simulink library "M160_lib"  (Simulink 7.8)
settings: Solver=FixedStepDiscrete  StartTime=0.0  StopTime=10.0  RelTol=1e-3
PreLoadFcn:
  | update_path
undefined symbols (not defined in the file): Afr_atCool2facLambdaReqCorr_CUR_x, Afr_atCool2facLambdaReqCorr_CUR_y, Afr_atMani2facLambdaReqCorr_CUR_x, Afr_atMani2facLambdaReqCorr_CUR_y, Afr_facLambdaReqMan, Afr_facRatioMan, Afr_facStoich, Afr_flgLambdaReqOverride, Afr_flgRatioOverride, Afr_rpmEngSpdfacRelAir2facLambdaReqBase_MAP_x, Afr_rpmEngSpdfacRelAir2facLambdaReqBase_MAP_y, Afr_rpmEngSpdfacRelAir2facLambdaReqBase_MAP_z, Ais_flgAirInjReacPumpOverride, Ais_stAirInjReacPumpMan, Amc_flgAirMassFlowOverride, Amc_uSens2AirMassFlow_CUR_x, Amc_uSens2AirMassFlow_CUR_y, Amc_uSensMaxValid, Amc_uSensMinValid, Amf_facRelAirMan, Amf_flgAirMassPerStrOverride, Amf_flgRelAirOverride, Amf_flgSwitch2AirMassFlowMeter, Amf_mAirPerStrMan, Amf_pManiEngSpd2facRelAirCorr_MAP_x, Amf_pManiEngSpd2facRelAirCorr_MAP_y, Amf_pManiEngSpd2facRelAirCorr_MAP_z, Amf_rpmEngSpd2facTempCorr_CUR_x, Amf_rpmEngSpd2facTempCorr_CUR_y, Amf_shcSpecGasConst_C, Amf_volEngDisp_C, Apv_facAirPumpRateMan, Apv_factor, Apv_flgAirPumpRateOverride, Apv_tiPeriod_C, Bvc_rVoltDivHigh, Bvc_rVoltDivLow, Bvc_uBattMax, Bvc_uBattMin, CDRV_E_OK_, Cov_facChOverVlvRateMan, Cov_factor, Cov_flgChOverVlvRateOverride, Cov_tiPeriod_C, Cpc_atManiTmp2facPresCorr_CUR_x, Cpc_atManiTmp2facPresCorr_CUR_y, Cpc_flgPChargeOverride, Cpc_uSens2pManiBase_CUR_x, Cpc_uSens2pManiBase_CUR_y, Ctc_rPullUp_C, Ctc_rSens2atCool_CUR_x, Ctc_rSens2atCool_CUR_y, Ctc_uSensMaxValid, Ctc_uSensMinValid, Ctc_uSupply, Doh_OutputDiagnosisOverride, dummy_facAirPumpRateReq, dummy_facChOverVlvRateReq, dummy_flgInterCoolerOverride, dummy_flgKl50Override ... (+243)
libraries: simulink x36, ehooks_lib x3
(part 2 of 8)

== system M160_lib/Actuators/Ivc ==
  Opm_idxMode : Inport
  Itc_flgInjCutoff : Inport  Port=2
  Itc_tiInj : Inport  Port=3
  Itc_tiBattDelay : Inport  Port=4
  Ivc : Subsystem
      mask Type: Actuators
      mask Description: InjectionValve
      mask Display:
      | image(imread('InjectionValve.jpg'))
      | port_label('input',1,'Opm_idxMode')
      | port_label('input',2,'Itc_flgInjCutoff')
      | port_label('input',3,'Itc_tiInj')
      | port_label('input',4,'Itc_tiBattDelay')
      | port_label('output',1,'Ivc_flgError')
  Ivc_Diag : Subsystem
      mask Type: Actuators
      mask Description: InjectionValveDiagnose
      mask Display:
      | image(imread('InjectionValve.jpg'))
      | port_label('output',1,'Ivc_flgError')
  Ivc_Diag_set : ehooks_lib/Library Blocks/ECU_FcnCallTrigger_Source  Tag=ECU_FcnCallTrigger_Source  Description=|  ProcessName=BypEasyhooks_100ms_Pre_Proc  TaskPriority=0  TaskPeriod=1
      | [$SL_INT_DD 20060]
      | EHOOKS ECU asynchronous function-call trigger source block.
  Ivc_Error : Subsystem
      mask Type: Actuators
      mask Description: InjectionValveError
      mask Display:
      | image(imread('InjectionValve.jpg'))
      | port_label('output',1,'Ivc_flgError')
  Ivc_set : ehooks_lib/Library Blocks/ECU_FcnCallTrigger_Source  Tag=ECU_FcnCallTrigger_Source  Description=|  ProcessName=BypEasyhooks_S0_Pre_Proc  TaskPriority=0  TaskPeriod=1
      | [$SL_INT_DD 20060]
      | EHOOKS ECU asynchronous function-call trigger source block.
  Ivc_set_Error : ehooks_lib/Library Blocks/ECU_FcnCallTrigger_Source  Tag=ECU_FcnCallTrigger_Source  Description=|  ProcessName=BypEasyhooks_S0_Pre_Proc  TaskPriority=0  TaskPeriod=1
      | [$SL_INT_DD 20060]
      | EHOOKS ECU asynchronous function-call trigger source block.
  Ivc_flgError : Outport
  wires:
  Ivc_set/1 -> Ivc/Trigger
  Ivc_Diag_set/1 -> Ivc_Diag/Trigger
  Opm_idxMode/1 -> Ivc/1(Opm_idxMode)
  Itc_flgInjCutoff/1 -> Ivc/2(Itc_flgInjCutoff)
  Itc_tiInj/1 -> Ivc/3(Itc_tiInj)
  Itc_tiBattDelay/1 -> Ivc/4(Itc_tiBattDelay)
  Ivc_set_Error/1 -> Ivc_Error/Trigger
  Ivc/1(Ivc_flgError) -> Ivc_Error/1(Ivc)
  Ivc_Diag/1(Ivc_flgError) -> Ivc_Error/2(Ivc_Diag)
  Ivc_Error/1(Ivc_flgError) -> Ivc_flgError/1

== system M160_lib/Actuators/Mrs ==
  Opm_idxMode : Inport
  dummy_stMainRelais : Inport  Port=2
  function : TriggerPort  TriggerType=function-call
  Constant1 : Constant  Value=Mrs_flgMainRelaisOverride
  Constant2 : Constant  Value=Mrs_stMainRelaisMan
  Constant5 : Constant  Value=Normal
  Constant6 : Constant  OutDataTypeStr=boolean
  G1_DigOut_Ctrl : Subsystem  AncestorBlock=ehooks_medc17flex_G1_lib/Library Blocks/Basic_IO/Outputs/G1_DigOut_Ctrl  LoadFcn=ehooks_medc17flex_devlib_io_block('load');  InitFcn=ehooks_medc17flex_devlib_io_block('init');  StartFcn=ehooks_medc17flex_devlib_io_block('start');  StopFcn=ehooks_medc17flex_devlib_io_block('stop');  ClipboardFcn=ehooks_medc17flex_devlib_io_block('clipboard', 0); % Second argument just needed to indicate null block. See callback handler.  mask{ChannelName=O_S_MRLY}
      mask prompts: ChannelName "Channel name"
      mask init:
      | ehooks_medc17flex_devlib_io_block('mask_init');
      settings: AttributesFormatString=Channel name: '%<ChannelName>'  CopyFcn=ehooks_medc17flex_devlib_io_block('copy');  DeleteFcn=ehooks_medc17flex_devlib_io_block('delete');  UndoDeleteFcn=ehooks_medc17flex_devlib_io_block('undo_delete');  ModelCloseFcn=ehooks_medc17flex_devlib_io_block('model_close');  PreSaveFcn=ehooks_medc17flex_devlib_io_block('pre_save');  PostSaveFcn=ehooks_medc17flex_devlib_io_block('post_save');  NameChangeFcn=ehooks_medc17flex_devlib_io_block('name_change');  DestroyFcn=ehooks_medc17flex_devlib_io_block('destroy', 0); % Second argument just needed to indicate null block. See callback handler.  OpenFcn=ehooks_medc17flex_devlib_io_block('open');  CloseFcn=ehooks_medc17flex_devlib_io_block('close');  ParentCloseFcn=ehooks_medc17flex_devlib_io_block('parent_close');  MoveFcn=ehooks_medc17flex_devlib_io_block('move');
      mask StyleString: popup(<empty>|O_S_MRLY|O_S_RL09|O_S_RL14|O_S_RL29|O_S_RL30|O_S_RL31|O_S_RL33|O_S_RL34|O_S_RL35|O_S_RL41|O_S_RL43)
      mask Display: image(imread('Output_Digital.jpg'))
  G1_DigOut_GetError : Subsystem  AncestorBlock=ehooks_medc17flex_G1_lib/Library Blocks/Basic_IO/Outputs/G1_DigOut_GetError  LoadFcn=ehooks_medc17flex_devlib_io_block('load');  InitFcn=ehooks_medc17flex_devlib_io_block('init');  StartFcn=ehooks_medc17flex_devlib_io_block('start');  StopFcn=ehooks_medc17flex_devlib_io_block('stop');  ClipboardFcn=ehooks_medc17flex_devlib_io_block('clipboard', 0); % Second argument just needed to indicate null block. See callback handler.  mask{ChannelName=O_S_MRLY}
      mask prompts: ChannelName "Channel name"
      mask init:
      | ehooks_medc17flex_devlib_io_block('mask_init');
      settings: AttributesFormatString=Channel name: '%<ChannelName>'  CopyFcn=ehooks_medc17flex_devlib_io_block('copy');  DeleteFcn=ehooks_medc17flex_devlib_io_block('delete');  UndoDeleteFcn=ehooks_medc17flex_devlib_io_block('undo_delete');  ModelCloseFcn=ehooks_medc17flex_devlib_io_block('model_close');  PreSaveFcn=ehooks_medc17flex_devlib_io_block('pre_save');  PostSaveFcn=ehooks_medc17flex_devlib_io_block('post_save');  NameChangeFcn=ehooks_medc17flex_devlib_io_block('name_change');  DestroyFcn=ehooks_medc17flex_devlib_io_block('destroy', 0); % Second argument just needed to indicate null block. See callback handler.  OpenFcn=ehooks_medc17flex_devlib_io_block('open');  CloseFcn=ehooks_medc17flex_devlib_io_block('close');  ParentCloseFcn=ehooks_medc17flex_devlib_io_block('parent_close');  MoveFcn=ehooks_medc17flex_devlib_io_block('move');
      mask StyleString: popup(<empty>|O_S_MRLY|O_S_RL09|O_S_RL14|O_S_RL29|O_S_RL30|O_S_RL31|O_S_RL33|O_S_RL34|O_S_RL35|O_S_RL41|O_S_RL43)
      mask Display: image(imread('Output_Digital_Diagnosis.jpg'))
  Logical Operator1 : Logic  Operator=NOT  AllPortsSameDT=off  OutDataTypeStr=boolean
  Logical Operator2 : Logic  Operator=NOT  AllPortsSameDT=off  OutDataTypeStr=boolean
  Relational Operator : RelationalOperator  Operator===  OutDataTypeStr=boolean
  Switch1 : Switch  Threshold=1
  Switch2 : Switch  Threshold=1
  Mrs_stDiagnosis : Outport
  Mrs_flgError : Outport  Port=2
  wires:
  Constant6/1 -> Switch2/3
  Relational Operator/1 -> Switch2/2
  Constant5/1 -> Relational Operator/2
  Opm_idxMode/1 -> Relational Operator/1
  Switch1/1 -> Switch2/1
  dummy_stMainRelais/1 -> Switch1/3
  Constant2/1 -> Switch1/1
  Constant1/1 -> Switch1/2
  Logical Operator1/1 -> Mrs_flgError/1  "Mrs_flgError"
  G1_DigOut_GetError/1(status) -> Mrs_stDiagnosis/1  "Mrs_stDiagnosis"
  Switch2/1 -> Logical Operator2/1  "Mrs_stMainRelais"
  Logical Operator2/1 -> G1_DigOut_Ctrl/1(state)
  G1_DigOut_Ctrl/1(status) -> Logical Operator1/1

== system M160_lib/Actuators/Str ==
  Opm_idxMode : Inport
  Stc_stStarter : Inport  Port=2
  function : TriggerPort  TriggerType=function-call
  Constant1 : Constant  Value=Str_flgStarterOverride
  Constant2 : Constant  Value=Str_stStarterMan
  Constant5 : Constant  Value=Normal
  Constant6 : Constant  Value=0  OutDataTypeStr=boolean
  G1_DigOut_Ctrl : Subsystem  AncestorBlock=ehooks_medc17flex_G1_lib/Library Blocks/Basic_IO/Outputs/G1_DigOut_Ctrl  LoadFcn=ehooks_medc17flex_devlib_io_block('load');  InitFcn=ehooks_medc17flex_devlib_io_block('init');  StartFcn=ehooks_medc17flex_devlib_io_block('start');  StopFcn=ehooks_medc17flex_devlib_io_block('stop');  ClipboardFcn=ehooks_medc17flex_devlib_io_block('clipboard', 0); % Second argument just needed to indicate null block. See callback handler.  mask{ChannelName=O_S_RL34}
      mask prompts: ChannelName "Channel name"
      mask init:
      | ehooks_medc17flex_devlib_io_block('mask_init');
      settings: AttributesFormatString=Channel name: '%<ChannelName>'  CopyFcn=ehooks_medc17flex_devlib_io_block('copy');  DeleteFcn=ehooks_medc17flex_devlib_io_block('delete');  UndoDeleteFcn=ehooks_medc17flex_devlib_io_block('undo_delete');  ModelCloseFcn=ehooks_medc17flex_devlib_io_block('model_close');  PreSaveFcn=ehooks_medc17flex_devlib_io_block('pre_save');  PostSaveFcn=ehooks_medc17flex_devlib_io_block('post_save');  NameChangeFcn=ehooks_medc17flex_devlib_io_block('name_change');  DestroyFcn=ehooks_medc17flex_devlib_io_block('destroy', 0); % Second argument just needed to indicate null block. See callback handler.  OpenFcn=ehooks_medc17flex_devlib_io_block('open');  CloseFcn=ehooks_medc17flex_devlib_io_block('close');  ParentCloseFcn=ehooks_medc17flex_devlib_io_block('parent_close');  MoveFcn=ehooks_medc17flex_devlib_io_block('move');
      mask StyleString: popup(<empty>|O_S_MRLY|O_S_RL09|O_S_RL14|O_S_RL29|O_S_RL30|O_S_RL31|O_S_RL33|O_S_RL34|O_S_RL35|O_S_RL41|O_S_RL43)
      mask Display: image(imread('Output_Digital.jpg'))
  G1_DigOut_GetError : Subsystem  AncestorBlock=ehooks_medc17flex_G1_lib/Library Blocks/Basic_IO/Outputs/G1_DigOut_GetError  LoadFcn=ehooks_medc17flex_devlib_io_block('load');  InitFcn=ehooks_medc17flex_devlib_io_block('init');  StartFcn=ehooks_medc17flex_devlib_io_block('start');  StopFcn=ehooks_medc17flex_devlib_io_block('stop');  ClipboardFcn=ehooks_medc17flex_devlib_io_block('clipboard', 0); % Second argument just needed to indicate null block. See callback handler.  mask{ChannelName=O_S_RL34}
      mask prompts: ChannelName "Channel name"
      mask init:
      | ehooks_medc17flex_devlib_io_block('mask_init');
      settings: AttributesFormatString=Channel name: '%<ChannelName>'  CopyFcn=ehooks_medc17flex_devlib_io_block('copy');  DeleteFcn=ehooks_medc17flex_devlib_io_block('delete');  UndoDeleteFcn=ehooks_medc17flex_devlib_io_block('undo_delete');  ModelCloseFcn=ehooks_medc17flex_devlib_io_block('model_close');  PreSaveFcn=ehooks_medc17flex_devlib_io_block('pre_save');  PostSaveFcn=ehooks_medc17flex_devlib_io_block('post_save');  NameChangeFcn=ehooks_medc17flex_devlib_io_block('name_change');  DestroyFcn=ehooks_medc17flex_devlib_io_block('destroy', 0); % Second argument just needed to indicate null block. See callback handler.  OpenFcn=ehooks_medc17flex_devlib_io_block('open');  CloseFcn=ehooks_medc17flex_devlib_io_block('close');  ParentCloseFcn=ehooks_medc17flex_devlib_io_block('parent_close');  MoveFcn=ehooks_medc17flex_devlib_io_block('move');
      mask StyleString: popup(<empty>|O_S_MRLY|O_S_RL09|O_S_RL14|O_S_RL29|O_S_RL30|O_S_RL31|O_S_RL33|O_S_RL34|O_S_RL35|O_S_RL41|O_S_RL43)
      mask Display: image(imread('Output_Digital_Diagnosis.jpg'))
  Logical Operator1 : Logic  Operator=NOT  AllPortsSameDT=off  OutDataTypeStr=boolean
  Logical Operator2 : Logic  Operator=NOT  AllPortsSameDT=off  OutDataTypeStr=boolean
  Relational Operator : RelationalOperator  Operator===  OutDataTypeStr=boolean
  Switch1 : Switch  Threshold=1
  Switch2 : Switch  Threshold=1
  Str_stDiagnosis : Outport
  Str_flgError : Outport  Port=2
  wires:
  Constant6/1 -> Switch2/3
  Relational Operator/1 -> Switch2/2
  Constant5/1 -> Relational Operator/2
  Opm_idxMode/1 -> Relational Operator/1
  Switch1/1 -> Switch2/1
  Stc_stStarter/1 -> Switch1/3
  Constant2/1 -> Switch1/1
  Constant1/1 -> Switch1/2
  Logical Operator1/1 -> Str_flgError/1  "Str_flgError"
  G1_DigOut_GetError/1(status) -> Str_stDiagnosis/1  "Str_stDiagnosis"
  Switch2/1 -> Logical Operator2/1  "Str_stStarter"
  Logical Operator2/1 -> G1_DigOut_Ctrl/1(state)
  G1_DigOut_Ctrl/1(status) -> Logical Operator1/1

== system M160_lib/Actuators/Tvc ==
  Opm_idxMode : Inport
  dummy_facThrValveReq : Inport  Port=2
  function : TriggerPort  TriggerType=function-call
  Bus Creator : BusCreator  Inputs=3
  Bus Selector : BusSelector  OutputSignals=Tvc_flgPosError,Tvc_facThrValveReq,Tvc_facThrValve
  Constant1 : Constant  Value=Tvc_flgThrValveReqOverride
  Constant2 : Constant  Value=Tvc_facThrValveReqMan
  Constant3 : Constant  Value=Tvc_facThrValveLimitMax
  Constant4 : Constant  Value=Tvc_facThrValveLimitMin
  Constant5 : Constant  Value=Normal
  Constant6 : Constant  Value=0.0  OutDataTypeStr=single
  Limiter : Subsystem
      mask Description: Limiter
      mask Display: image(imread('Limiter.jpg'))
  Logical Operator : Logic  Operator=OR  AllPortsSameDT=off  OutDataTypeStr=boolean
  Logical Operator1 : Logic  Operator=NOT  AllPortsSameDT=off  OutDataTypeStr=boolean
  Relational Operator : RelationalOperator  Operator===  OutDataTypeStr=boolean
  Switch1 : Switch  Threshold=1
  Switch2 : Switch  Threshold=1
  ThrottleValveControl : Subsystem
  ThrottleValveOutput : Subsystem
  ThrottleValvePosition : Subsystem
  Tvc_stDiagnosis : Outport
  Tvc_flgError : Outport  Port=2
  tag scope: Opm_idxMode_global=global
  wires:
  ThrottleValvePosition/1(Tvc_flgPosError) -> Bus Creator/1  "Tvc_flgPosError"
  ThrottleValvePosition/2(Tvc_facThrValve) -> Bus Creator/2  "Tvc_facThrValve"
  Bus Creator/1 -> Bus Selector/1
  Bus Selector/1 -> Logical Operator/1, ThrottleValveOutput/1(Tvc_flgPosError), ThrottleValveControl/1(Tvc_flgPosError)  "<Tvc_flgPosError>"
  Logical Operator1/1 -> Logical Operator/2
  ThrottleValveOutput/1(Tvc_stHBridge) -> Logical Operator1/1
  ThrottleValveControl/1(Tvc_facDutycycle) -> ThrottleValveOutput/2(Tvc_facDutycycle)  "Tvc_facDutycycle"
  Constant3/1 -> Limiter/1(max)
  Constant4/1 -> Limiter/3(min)
  dummy_facThrValveReq/1 -> Limiter/2(in)
  Constant1/1 -> Switch1/2
  Opm_idxMode/1 -> [Opm_idxMode_global], Relational Operator/1
  Constant5/1 -> Relational Operator/2
  Relational Operator/1 -> Switch2/2
  Switch1/1 -> Switch2/1
  Switch2/1 -> Bus Creator/3  "Tvc_facThrValveReq"
  Constant6/1 -> Switch2/3
  Logical Operator/1 -> Tvc_flgError/1  "Tvc_flgError"
  Bus Selector/2 -> ThrottleValveControl/2(Tvc_facThrValve)  "<Tvc_facThrValveReq>"
  Bus Selector/3 -> ThrottleValveControl/3(Tvc_facThrValveReq)  "<Tvc_facThrValve>"
  ThrottleValveOutput/2(Tvc_stDiagnosis) -> Tvc_stDiagnosis/1  "Tvc_stDiagnosis"
  Limiter/1(return) -> Switch1/3
  Constant2/1 -> Switch1/1

== system M160_lib/Actuators/Wcs ==
  Opm_idxMode : Inport
  Ctc_atCool : Inport  Port=2
  function : TriggerPort  TriggerType=function-call
  Constant1 : Constant  Value=Wcs_flgWaterCoolerOverride
  Constant2 : Constant  Value=Wcs_stWaterCoolerMan
  Constant5 : Constant  Value=Normal
  Constant6 : Constant  Value=0  OutDataTypeStr=boolean
  G1_DigOut_Ctrl : Subsystem  AncestorBlock=ehooks_medc17flex_G1_lib/Library Blocks/Basic_IO/Outputs/G1_DigOut_Ctrl  LoadFcn=ehooks_medc17flex_devlib_io_block('load');  InitFcn=ehooks_medc17flex_devlib_io_block('init');  StartFcn=ehooks_medc17flex_devlib_io_block('start');  StopFcn=ehooks_medc17flex_devlib_io_block('stop');  ClipboardFcn=ehooks_medc17flex_devlib_io_block('clipboard', 0); % Second argument just needed to indicate null block. See callback handler.  mask{ChannelName=O_S_RL14}
      mask prompts: ChannelName "Channel name"
      mask init:
      | ehooks_medc17flex_devlib_io_block('mask_init');
      settings: AttributesFormatString=Channel name: '%<ChannelName>'  CopyFcn=ehooks_medc17flex_devlib_io_block('copy');  DeleteFcn=ehooks_medc17flex_devlib_io_block('delete');  UndoDeleteFcn=ehooks_medc17flex_devlib_io_block('undo_delete');  ModelCloseFcn=ehooks_medc17flex_devlib_io_block('model_close');  PreSaveFcn=ehooks_medc17flex_devlib_io_block('pre_save');  PostSaveFcn=ehooks_medc17flex_devlib_io_block('post_save');  NameChangeFcn=ehooks_medc17flex_devlib_io_block('name_change');  DestroyFcn=ehooks_medc17flex_devlib_io_block('destroy', 0); % Second argument just needed to indicate null block. See callback handler.  OpenFcn=ehooks_medc17flex_devlib_io_block('open');  CloseFcn=ehooks_medc17flex_devlib_io_block('close');  ParentCloseFcn=ehooks_medc17flex_devlib_io_block('parent_close');  MoveFcn=ehooks_medc17flex_devlib_io_block('move');
      mask StyleString: popup(<empty>|O_S_MRLY|O_S_RL09|O_S_RL14|O_S_RL29|O_S_RL30|O_S_RL31|O_S_RL33|O_S_RL34|O_S_RL35|O_S_RL41|O_S_RL43)
      mask Display: image(imread('Output_Digital.jpg'))
  G1_DigOut_GetError : Subsystem  AncestorBlock=ehooks_medc17flex_G1_lib/Library Blocks/Basic_IO/Outputs/G1_DigOut_GetError  LoadFcn=ehooks_medc17flex_devlib_io_block('load');  InitFcn=ehooks_medc17flex_devlib_io_block('init');  StartFcn=ehooks_medc17flex_devlib_io_block('start');  StopFcn=ehooks_medc17flex_devlib_io_block('stop');  ClipboardFcn=ehooks_medc17flex_devlib_io_block('clipboard', 0); % Second argument just needed to indicate null block. See callback handler.  mask{ChannelName=O_S_RL14}
      mask prompts: ChannelName "Channel name"
      mask init:
      | ehooks_medc17flex_devlib_io_block('mask_init');
      settings: AttributesFormatString=Channel name: '%<ChannelName>'  CopyFcn=ehooks_medc17flex_devlib_io_block('copy');  DeleteFcn=ehooks_medc17flex_devlib_io_block('delete');  UndoDeleteFcn=ehooks_medc17flex_devlib_io_block('undo_delete');  ModelCloseFcn=ehooks_medc17flex_devlib_io_block('model_close');  PreSaveFcn=ehooks_medc17flex_devlib_io_block('pre_save');  PostSaveFcn=ehooks_medc17flex_devlib_io_block('post_save');  NameChangeFcn=ehooks_medc17flex_devlib_io_block('name_change');  DestroyFcn=ehooks_medc17flex_devlib_io_block('destroy', 0); % Second argument just needed to indicate null block. See callback handler.  OpenFcn=ehooks_medc17flex_devlib_io_block('open');  CloseFcn=ehooks_medc17flex_devlib_io_block('close');  ParentCloseFcn=ehooks_medc17flex_devlib_io_block('parent_close');  MoveFcn=ehooks_medc17flex_devlib_io_block('move');
      mask StyleString: popup(<empty>|O_S_MRLY|O_S_RL09|O_S_RL14|O_S_RL29|O_S_RL30|O_S_RL31|O_S_RL33|O_S_RL34|O_S_RL35|O_S_RL41|O_S_RL43)
      mask Display: image(imread('Output_Digital_Diagnosis.jpg'))
  Hysteresis_Delta_RSP : Subsystem
      mask Description: Hysteresis_Delta_RSP
      mask Display: image(imread('HysteresDeltaR.jpg'))
  Logical Operator1 : Logic  Operator=NOT  AllPortsSameDT=off  OutDataTypeStr=boolean
  Logical Operator2 : Logic  Operator=NOT  AllPortsSameDT=off  OutDataTypeStr=boolean
  Relational Operator : RelationalOperator  Operator===  OutDataTypeStr=boolean
  Switch1 : Switch  Threshold=1
  Switch2 : Switch  Threshold=1
  Wcs_stDiagnosis : Outport
  Wcs_flgError : Outport  Port=2
  wires:
  Constant6/1 -> Switch2/3
  Relational Operator/1 -> Switch2/2
  Constant5/1 -> Relational Operator/2
  Opm_idxMode/1 -> Relational Operator/1
  Switch1/1 -> Switch2/1
  Ctc_atCool/1 -> Hysteresis_Delta_RSP/1(in)
  Constant2/1 -> Switch1/1
  Constant1/1 -> Switch1/2
  Logical Operator1/1 -> Wcs_flgError/1  "Wcs_flgError"
  G1_DigOut_GetError/1(status) -> Wcs_stDiagnosis/1  "Wcs_stDiagnosis"
  Switch2/1 -> Logical Operator2/1  "Wcs_stWaterCooler"
  Logical Operator2/1 -> G1_DigOut_Ctrl/1(state)
  G1_DigOut_Ctrl/1(status) -> Logical Operator1/1
  Hysteresis_Delta_RSP/1(return) -> Switch1/3

== system M160_lib/Actuators/Wgc ==
  Opm_idxMode : Inport
  T2t_facWasteGateRate : Inport  Port=2
  function : TriggerPort  TriggerType=function-call
  Constant1 : Constant  Value=Wgc_flgWastegateRateOverride
  Constant2 : Constant  Value=Wgc_facWasteGateRateMan
  Constant3 : Constant  Value=10000  OutDataTypeStr=single
  Constant4 : Constant  Value=Wgc_factor
  Constant5 : Constant  Value=Normal
  Constant6 : Constant  Value=0.0  OutDataTypeStr=single
  Constant7 : Constant  Value=Wgc_tiPeriod_C
  Constant9 : Constant  Value=Lo_
  G1_PWM_Output_Ctrl : Subsystem  AncestorBlock=ehooks_medc17flex_G1_lib/Library Blocks/Basic_IO/Outputs/G1_PWM_Output_Ctrl  LoadFcn=ehooks_medc17flex_devlib_io_block('load');  InitFcn=ehooks_medc17flex_devlib_io_block('init');  StartFcn=ehooks_medc17flex_devlib_io_block('start');  StopFcn=ehooks_medc17flex_devlib_io_block('stop');  ClipboardFcn=ehooks_medc17flex_devlib_io_block('clipboard', 0); % Second argument just needed to indicate null block. See callback handler.  mask{ChannelName=O_T_RL22}
      mask prompts: ChannelName "Channel name"
      mask init:
      | ehooks_medc17flex_devlib_io_block('mask_init');
      settings: AttributesFormatString=Channel name: '%<ChannelName>'  CopyFcn=ehooks_medc17flex_devlib_io_block('copy');  DeleteFcn=ehooks_medc17flex_devlib_io_block('delete');  UndoDeleteFcn=ehooks_medc17flex_devlib_io_block('undo_delete');  ModelCloseFcn=ehooks_medc17flex_devlib_io_block('model_close');  PreSaveFcn=ehooks_medc17flex_devlib_io_block('pre_save');  PostSaveFcn=ehooks_medc17flex_devlib_io_block('post_save');  NameChangeFcn=ehooks_medc17flex_devlib_io_block('name_change');  DestroyFcn=ehooks_medc17flex_devlib_io_block('destroy', 0); % Second argument just needed to indicate null block. See callback handler.  OpenFcn=ehooks_medc17flex_devlib_io_block('open');  CloseFcn=ehooks_medc17flex_devlib_io_block('close');  ParentCloseFcn=ehooks_medc17flex_devlib_io_block('parent_close');  MoveFcn=ehooks_medc17flex_devlib_io_block('move');
      mask StyleString: popup(<empty>|O_T_RL10|O_T_RL13|O_T_RL19|O_T_RL20|O_T_RL22|O_T_RL23|O_T_RL25|O_T_RL26|O_T_RL27|O_T_RL28|O_T_RL38|O_T_RL39|O_T_RL40|O_T_RL42|O_T_RL44|O_T_RL45|O_T_RL46|O_T_RL47|O_T_RL48|O_T_RL49|O_T_RL50|O_T_RH02)
      mask Display: image(imread('Output_PWM.jpg'))
  G1_PwmOut_Get_error : Subsystem  AncestorBlock=ehooks_medc17flex_G1_lib/Library Blocks/Basic_IO/Outputs/G1_PwmOut_Get_error  LoadFcn=ehooks_medc17flex_devlib_io_block('load');  InitFcn=ehooks_medc17flex_devlib_io_block('init');  StartFcn=ehooks_medc17flex_devlib_io_block('start');  StopFcn=ehooks_medc17flex_devlib_io_block('stop');  ClipboardFcn=ehooks_medc17flex_devlib_io_block('clipboard', 0); % Second argument just needed to indicate null block. See callback handler.  mask{ChannelName=O_T_RL22}
      mask prompts: ChannelName "Channel name"
      mask init:
      | ehooks_medc17flex_devlib_io_block('mask_init');
      settings: AttributesFormatString=Channel name: '%<ChannelName>'  CopyFcn=ehooks_medc17flex_devlib_io_block('copy');  DeleteFcn=ehooks_medc17flex_devlib_io_block('delete');  UndoDeleteFcn=ehooks_medc17flex_devlib_io_block('undo_delete');  ModelCloseFcn=ehooks_medc17flex_devlib_io_block('model_close');  PreSaveFcn=ehooks_medc17flex_devlib_io_block('pre_save');  PostSaveFcn=ehooks_medc17flex_devlib_io_block('post_save');  NameChangeFcn=ehooks_medc17flex_devlib_io_block('name_change');  DestroyFcn=ehooks_medc17flex_devlib_io_block('destroy', 0); % Second argument just needed to indicate null block. See callback handler.  OpenFcn=ehooks_medc17flex_devlib_io_block('open');  CloseFcn=ehooks_medc17flex_devlib_io_block('close');  ParentCloseFcn=ehooks_medc17flex_devlib_io_block('parent_close');  MoveFcn=ehooks_medc17flex_devlib_io_block('move');
      mask StyleString: popup(<empty>|O_T_RL10|O_T_RL13|O_T_RL19|O_T_RL20|O_T_RL22|O_T_RL23|O_T_RL25|O_T_RL26|O_T_RL27|O_T_RL28|O_T_RL38|O_T_RL39|O_T_RL40|O_T_RL42|O_T_RL44|O_T_RL45|O_T_RL46|O_T_RL47|O_T_RL48|O_T_RL49|O_T_RL50|O_T_RH02)
      mask Display: image(imread('Output_PWM_Diagnosis.jpg'))
  Logical Operator1 : Logic  Operator=NOT  AllPortsSameDT=off  OutDataTypeStr=boolean
  Product1 : Product  OutDataTypeStr=Inherit: Same as first input
  Relational Operator : RelationalOperator  Operator===  OutDataTypeStr=boolean
  Switch1 : Switch  Threshold=1
  Switch2 : Switch  Threshold=1
  Fps_stDiagnosis : Outport
  Fps_flgError : Outport  Port=2
  wires:
  Constant6/1 -> Switch2/3
  Relational Operator/1 -> Switch2/2
  Constant5/1 -> Relational Operator/2
  Opm_idxMode/1 -> Relational Operator/1
  Switch1/1 -> Switch2/1
  T2t_facWasteGateRate/1 -> Switch1/3
  Constant2/1 -> Switch1/1
  Constant1/1 -> Switch1/2
  Logical Operator1/1 -> Fps_flgError/1  "Wgc_flgError"
  G1_PwmOut_Get_error/1(status) -> Fps_stDiagnosis/1  "Wgc_stDiagnosis"
  Switch2/1 -> Product1/1  "Wgc_facWasteGateRate"
  G1_PWM_Output_Ctrl/1(status) -> Logical Operator1/1
  Constant3/1 -> Product1/2
  Product1/1 -> G1_PWM_Output_Ctrl/1(dutycycle)
  Constant7/1 -> G1_PWM_Output_Ctrl/2(period)
  Constant4/1 -> G1_PWM_Output_Ctrl/3(factor)
  Constant9/1 -> G1_PWM_Output_Ctrl/4(level)

== system M160_lib/Functions/Afr ==
  Epm_rpmEngSpd : Inport
  Mtc_atMani : Inport  Port=2
  Ctc_atCool : Inport  Port=3
  Amf_facRelAir : Inport  Port=4
  function : TriggerPort  TriggerType=function-call
  Afr_atCool2facLambdaReqCorr_CUR : Lookup_n-D  NumberOfTableDimensions=1  BreakpointsForDimension1=Afr_atCool2facLambdaReqCorr_CUR_x  Table=Afr_atCool2facLambdaReqCorr_CUR_y  ExtrapMethod=Clip  InputSameDT=on
  Afr_atMani2facLambdaReqCorr_CUR : Lookup_n-D  NumberOfTableDimensions=1  BreakpointsForDimension1=Afr_atMani2facLambdaReqCorr_CUR_x  Table=Afr_atMani2facLambdaReqCorr_CUR_y  ExtrapMethod=Clip  InputSameDT=on
  Afr_rpmEngSpdfacRelAir2facLambdaReqBase_MAP : Lookup_n-D  BreakpointsForDimension1=Afr_rpmEngSpdfacRelAir2facLambdaReqBase_MAP_x  BreakpointsForDimension2=Afr_rpmEngSpdfacRelAir2facLambdaReqBase_MAP_y  Table=Afr_rpmEngSpdfacRelAir2facLambdaReqBase_MAP_z  ExtrapMethod=Clip  InputSameDT=on
  Constant1 : Constant  Value=Afr_flgLambdaReqOverride
  Constant2 : Constant  Value=Afr_flgRatioOverride
  Constant3 : Constant  Value=Afr_facLambdaReqMan
  Constant4 : Constant  Value=Afr_facRatioMan
  Constant5 : Constant  Value=Afr_facStoich
  Product2 : Product  OutDataTypeStr=Inherit: Same as first input
  Subtract : Sum  OutDataTypeStr=Inherit: Same as first input
  Subtract1 : Sum  OutDataTypeStr=Inherit: Same as first input
  Switch1 : Switch  Threshold=1
  Switch2 : Switch  Threshold=1
  Afr_facLambdaReq : Outport
  Afr_facRatio : Outport  Port=2
  wires:
  Epm_rpmEngSpd/1 -> Afr_rpmEngSpdfacRelAir2facLambdaReqBase_MAP/1
  Amf_facRelAir/1 -> Afr_rpmEngSpdfacRelAir2facLambdaReqBase_MAP/2
  Afr_rpmEngSpdfacRelAir2facLambdaReqBase_MAP/1 -> Subtract/1
  Subtract/1 -> Subtract1/1
  Ctc_atCool/1 -> Afr_atCool2facLambdaReqCorr_CUR/1
  Afr_atCool2facLambdaReqCorr_CUR/1 -> Subtract/2
  Mtc_atMani/1 -> Afr_atMani2facLambdaReqCorr_CUR/1
  Afr_atMani2facLambdaReqCorr_CUR/1 -> Subtract1/2
  Subtract1/1 -> Switch1/3, Product2/1  "Afr_facLambdaReqCalc"
  Constant1/1 -> Switch1/2
  Constant3/1 -> Switch1/1
  Switch1/1 -> Afr_facLambdaReq/1  "Afr_facLambdaReq"
  Switch2/1 -> Afr_facRatio/1  "Afr_facRatio"
  Product2/1 -> Switch2/3  "Afr_facRatioCalc"
  Constant5/1 -> Product2/2
  Constant2/1 -> Switch2/2
  Constant4/1 -> Switch2/1

== system M160_lib/Functions/Amf ==
  note: Pa/(K*(J/(K*kg))) = (N/m^2)/(K*(N*m/(K*kg))) = kg/m^3
  note: cm^3*kg/m^3 = 10^-6*m^3*10^3*g/m^3 = 10^-3*g
  note: 1000 g/kg - Umrechnung in kg
      | 2 - 2 Umdrehungen pro Arbeitsspiel
  note: umrechung Drehzahl in 1/h
  note: 1000 g/kg - Umrechnung in kg
      | 2 - 2 Umdrehungen pro Arbeitsspiel
  Epm_rpmEngSpd : Inport
  Mtc_atMani : Inport  Port=2
  Mpc_pManiFilt : Inport  Port=3
  Ctc_atCool : Inport  Port=4
  Amc_AirMassFlow : Inport  Port=5
  function : TriggerPort  TriggerType=function-call
  Amf_mAirCalc : Terminator
  Amf_pManiEngSpd2facRelAirCorr_MAP : Lookup_n-D  BreakpointsForDimension1=Amf_pManiEngSpd2facRelAirCorr_MAP_x  BreakpointsForDimension2=Amf_pManiEngSpd2facRelAirCorr_MAP_y  Table=Amf_pManiEngSpd2facRelAirCorr_MAP_z  ExtrapMethod=Clip  InputSameDT=on
  Amf_rpmEngSpd2facTempCorr_CUR : Lookup_n-D  NumberOfTableDimensions=1  BreakpointsForDimension1=Amf_rpmEngSpd2facTempCorr_CUR_x  Table=Amf_rpmEngSpd2facTempCorr_CUR_y  ExtrapMethod=Clip  InputSameDT=on
  Constan1 : Constant  Value=273  OutDataTypeStr=single
  Constan2 : Constant  Value=273  OutDataTypeStr=single
  Constan3 : Constant  Value=101300  OutDataTypeStr=single
  Constan4 : Constant  Value=0.001  OutMin=0  OutDataTypeStr=single
  Constan5 : Constant  Value=3  OutDataTypeStr=single
  Constan6 : Constant  Value=2000  OutDataTypeStr=single
  Constan7 : Constant  Value=3  OutDataTypeStr=single
  Constan8 : Constant  Value=60  OutDataTypeStr=single
  Constan9 : Constant  Value=2000  OutDataTypeStr=single
  Constant1 : Constant  Value=Amf_volEngDisp_C
  Constant2 : Constant  Value=Amf_shcSpecGasConst_C
  Constant3 : Constant  Value=Amf_facRelAirMan
  Constant4 : Constant  Value=Amf_flgSwitch2AirMassFlowMeter
  Constant5 : Constant  Value=Amf_flgRelAirOverride
  Constant6 : Constant  Value=Amf_mAirPerStrMan
  Constant7 : Constant  Value=Amf_flgAirMassPerStrOverride
  Divide{,1..5} (6 alike) : Product  Inputs=*/  OutDataTypeStr=Inherit: Same as first input
  Product{,1..3,7} (5 alike) : Product  OutDataTypeStr=Inherit: Same as first input
  Product4 : Product  Inputs=3  OutDataTypeStr=Inherit: Same as first input
  Product5 : Product  Inputs=4  OutDataTypeStr=Inherit: Same as first input
  Product6 : Product  Inputs=3  OutDataTypeStr=Inherit: Same as first input
  Subtract : Sum  OutDataTypeStr=Inherit: Same as first input
  Subtract1 : Sum  Inputs=+-  OutDataTypeStr=Inherit: Same as first input
  Switch{1..4} (4 alike) : Switch  Threshold=1
  Amf_mAirPerStr : Outport
  Amf_facRelAir : Outport  Port=2
  wires:
  Epm_rpmEngSpd/1 -> Amf_pManiEngSpd2facRelAirCorr_MAP/2, Amf_rpmEngSpd2facTempCorr_CUR/1, Divide3/1
  Mpc_pManiFilt/1 -> Amf_pManiEngSpd2facRelAirCorr_MAP/1
  Amf_rpmEngSpd2facTempCorr_CUR/1 -> Product/1
  Product/1 -> Subtract/1
  Ctc_atCool/1 -> Subtract1/1
  Mtc_atMani/1 -> Subtract1/2, Subtract/2
  Subtract1/1 -> Product/2
  Constan2/1 -> Divide/1
  Subtract/1 -> Divide/2  "Amf_atAirIntake"
  Constan3/1 -> Divide1/1
  Constan1/1 -> Product1/1
  Product1/1 -> Divide1/2
  Constant2/1 -> Product1/2
  Divide/1 -> Product2/2  "Amf_facRelAirTempCorr"
  Amf_pManiEngSpd2facRelAirCorr_MAP/1 -> Product2/1  "Amf_facRelAirBase"
  Divide1/1 -> Product4/2  "Amf_rohAirDen"
  Constant1/1 -> Divide2/1
  Constan5/1 -> Divide2/2
  Constan4/1 -> Product4/1
  Divide2/1 -> Product4/3
  Product2/1 -> Product3/1, Switch2/3  "Amf_facRelAirCalc"
  Product4/1 -> Product3/2, Divide5/2  "Amf_facMRelAir100"
  Switch2/1 -> Switch1/3
  Constant5/1 -> Switch2/2
  Constant3/1 -> Switch2/1
  Switch1/1 -> Amf_facRelAir/1  "Amf_facRelAir"
  Constant4/1 -> Switch1/2, Switch4/2
  Constant7/1 -> Switch3/2
  Constant6/1 -> Switch3/1
  Product3/1 -> Switch3/3  "Amf_mAirPerStrCalc"
  Switch3/1 -> Switch4/3
  Switch4/1 -> Amf_mAirPerStr/1, Product5/1  "Amf_mAirPerStr"
  Constan6/1 -> Divide3/2
  Product5/1 -> Amf_mAirCalc/1  "Amf_mAirCalc"
  Divide3/1 -> Product5/2, Product6/3
  Constan7/1 -> Product5/3, Product6/2
  Constan8/1 -> Product5/4, Product6/1
  Amc_AirMassFlow/1 -> Product7/1
  Constan9/1 -> Product7/2
  Product7/1 -> Divide4/1
  Product6/1 -> Divide4/2
  Divide4/1 -> Divide5/1, Switch4/1  "Amf_mAirPerStroke_AirMassFlowMeter"
  Divide5/1 -> Switch1/1  "Amf_facRelAir_AirMassFlowMeter"

== system M160_lib/Functions/Doh ==
  In1 : Inport
  In2 : Inport  Port=2
  In3 : Inport  Port=3
  In4 : Inport  Port=4
  In5 : Inport  Port=5
  In6 : Inport  Port=6
  In7 : Inport  Port=7
  In8 : Inport  Port=8
  In9 : Inport  Port=9
  In10 : Inport  Port=10
  function : TriggerPort  TriggerType=function-call
  Constant1 : Constant  Value=Doh_OutputDiagnosisOverride
  Constant6 : Constant  Value=0  OutDataTypeStr=boolean
  DiagnosisOutput_1 : Subsystem
  DiagnosisOutput_10 : Subsystem
  DiagnosisOutput_2 : Subsystem
  DiagnosisOutput_3 : Subsystem
  DiagnosisOutput_4 : Subsystem
  DiagnosisOutput_5 : Subsystem
  DiagnosisOutput_6 : Subsystem
  DiagnosisOutput_7 : Subsystem
  DiagnosisOutput_8 : Subsystem
  DiagnosisOutput_9 : Subsystem
  Logical Operator4 : Logic  Operator=OR  Inputs=10  AllPortsSameDT=off  OutDataTypeStr=boolean
  Switch2 : Switch  Threshold=1
  Doh_flgErrorDiagnosis : Outport
  wires:
  Constant1/1 -> Switch2/2
  Switch2/1 -> Doh_flgErrorDiagnosis/1  "Doh_flgErrorDiagnosis"
  Constant6/1 -> Switch2/1
  Logical Operator4/1 -> Switch2/3
  In1/1 -> DiagnosisOutput_1/1(status)
  DiagnosisOutput_1/1(stError) -> Logical Operator4/1
  In2/1 -> DiagnosisOutput_2/1(status)
  DiagnosisOutput_2/1(stError) -> Logical Operator4/2
  In3/1 -> DiagnosisOutput_3/1(status)
  DiagnosisOutput_3/1(stError) -> Logical Operator4/3
  In4/1 -> DiagnosisOutput_4/1(status)
  DiagnosisOutput_4/1(stError) -> Logical Operator4/4
  In5/1 -> DiagnosisOutput_5/1(status)
  DiagnosisOutput_5/1(stError) -> Logical Operator4/5
  In6/1 -> DiagnosisOutput_6/1(status)
  DiagnosisOutput_6/1(stError) -> Logical Operator4/6
  In7/1 -> DiagnosisOutput_7/1(status)
  DiagnosisOutput_7/1(stError) -> Logical Operator4/7
  In8/1 -> DiagnosisOutput_8/1(status)
  DiagnosisOutput_8/1(stError) -> Logical Operator4/8
  In9/1 -> DiagnosisOutput_9/1(status)
  DiagnosisOutput_9/1(stError) -> Logical Operator4/9
  In10/1 -> DiagnosisOutput_10/1(status)
  DiagnosisOutput_10/1(stError) -> Logical Operator4/10

== system M160_lib/Functions/Dummy ==
  T2t_facThrValveReq : Inport
  Egc_facEgas : Inport  Port=2
  Epm_rpmEngSpd : Inport  Port=3
  ICC_flgInterCooler : Inport  Port=4
  Kl50_stKlemme50 : Inport  Port=5
  function : TriggerPort  TriggerType=function-call
  Constant1 : Constant  Value=dummy_flgT2tOverride
  Constant10 : Constant  Value=dummy_flgKl50Override
  Constant11 : Constant  Value=dummy_StarterReq
  Constant2 : Constant  Value=dummy_facAirPumpRateReq
  Constant3 : Constant  Value=dummy_facChOverVlvRateReq
  Constant4 : Constant  Value=dummy_stMainRelaisReq
  Constant5 : Constant  Value=dummy_stFuelPumpReq
  Constant6 : Constant  Value=dummy_rpmFuelPumpMin
  Constant7 : Constant  Value=dummy_flgInterCoolerOverride
  Constant8 : Constant  Value=dummy_stIntercoolerReq
  Constant9 : Constant  Value=dummy_stAirInjReacPumpReq
  Logical Operator2 : Logic  AllPortsSameDT=off  OutDataTypeStr=boolean
  Relational Oprator2 : RelationalOperator  Operator=>  OutDataTypeStr=boolean
  Switch1 : Switch  Threshold=1
  Switch2 : Switch  Threshold=1
  Switch4 : Switch  Threshold=1
  dummy_facThrValveReq : Outport
  dummy_facAirPumpRate : Outport  Port=2
  dummy_facChOverVlvRate : Outport  Port=3
  dummy_stMainRelais : Outport  Port=4
  dummy_stFuelPump : Outport  Port=5
  dummy_stIntercooler : Outport  Port=6
  dummy_stAirInjReacPump : Outport  Port=7
  dummy_Starter : Outport  Port=8
  wires:
  Egc_facEgas/1 -> Switch4/1
  Constant1/1 -> Switch4/2
  T2t_facThrValveReq/1 -> Switch4/3
  Switch4/1 -> dummy_facThrValveReq/1  "dummy_facThrValveReq"
  Constant2/1 -> dummy_facAirPumpRate/1  "dummy_facAirPumpRate"
  Constant3/1 -> dummy_facChOverVlvRate/1  "dummy_facChOverVlvRate"
  Constant4/1 -> dummy_stMainRelais/1  "dummy_stMainRelais"
  Epm_rpmEngSpd/1 -> Relational Oprator2/1
  Relational Oprator2/1 -> Logical Operator2/2
  Constant5/1 -> Logical Operator2/1
  Logical Operator2/1 -> dummy_stFuelPump/1  "dummy_stFuelPump"
  Constant6/1 -> Relational Oprator2/2
  Constant7/1 -> Switch1/2
  Constant8/1 -> Switch1/1
  ICC_flgInterCooler/1 -> Switch1/3
  Switch1/1 -> dummy_stIntercooler/1  "dummy_stIntercooler"
  Constant9/1 -> dummy_stAirInjReacPump/1  "dummy_stAirInjReacPump"
  Kl50_stKlemme50/1 -> Switch2/3
  Constant11/1 -> Switch2/1
  Constant10/1 -> Switch2/2
  Switch2/1 -> dummy_Starter/1  "dummy_Starter"

== system M160_lib/Functions/Eih ==
  In1 : Inport
  In2 : Inport  Port=2
  In3 : Inport  Port=3
  In4 : Inport  Port=4
  In5 : Inport  Port=5
  In6 : Inport  Port=6
  In7 : Inport  Port=7
  In8 : Inport  Port=8
  In9 : Inport  Port=9
  function : TriggerPort  TriggerType=function-call
  Logical Operator4 : Logic  Operator=OR  Inputs=9  AllPortsSameDT=off  OutDataTypeStr=boolean
  Eih_flgInputError : Outport
  wires:
  Logical Operator4/1 -> Eih_flgInputError/1  "Eih_flgInputError"
  In1/1 -> Logical Operator4/1
  In2/1 -> Logical Operator4/2
  In3/1 -> Logical Operator4/3
  In4/1 -> Logical Operator4/4
  In5/1 -> Logical Operator4/5
  In6/1 -> Logical Operator4/6
  In7/1 -> Logical Operator4/7
  In8/1 -> Logical Operator4/8
  In9/1 -> Logical Operator4/9

== system M160_lib/Functions/Eoh ==
  In1 : Inport
  In2 : Inport  Port=2
  In3 : Inport  Port=3
  In4 : Inport  Port=4
  In5 : Inport  Port=5
  In6 : Inport  Port=6
  In7 : Inport  Port=7
  In8 : Inport  Port=8
  In9 : Inport  Port=9
  In10 : Inport  Port=10
  In11 : Inport  Port=11
  In12 : Inport  Port=12
  function : TriggerPort  TriggerType=function-call
  Logical Operator4 : Logic  Operator=OR  Inputs=12  AllPortsSameDT=off  OutDataTypeStr=boolean
  Eoh_flgOutputError : Outport
  wires:
  Logical Operator4/1 -> Eoh_flgOutputError/1  "Eoh_flgOutputError"
  In1/1 -> Logical Operator4/1
  In2/1 -> Logical Operator4/2
  In3/1 -> Logical Operator4/3
  In4/1 -> Logical Operator4/4
  In5/1 -> Logical Operator4/5
  In6/1 -> Logical Operator4/6
  In7/1 -> Logical Operator4/7
  In8/1 -> Logical Operator4/8
  In9/1 -> Logical Operator4/9
  In10/1 -> Logical Operator4/10
  In11/1 -> Logical Operator4/11
  In12/1 -> Logical Operator4/12

== system M160_lib/Functions/Fmc ==
  note: FuelMass per Stroke * 3 Cylinders * 60 min/h / (Torque * pi / 30 / 1000)
  Epm_rpmEngSpd : Inport
  Lcc_facLambdaCorr : Inport  Port=2
  Afr_facRatio : Inport  Port=3
  Amf_mAirPerStr : Inport  Port=4
  Tqs_tqReq : Inport  Port=5
  Itc_tiInjOffset : Inport  Port=6
  function : TriggerPort  TriggerType=function-call
  Constan1 : Constant  OutDataTypeStr=single
  Constan10 : Constant  Value=2000  OutDataTypeStr=single
  Constan11 : Constant  Value=3.141  OutDataTypeStr=single
  Constan12 : Constant  Value=2  OutDataTypeStr=single
  Constan2 : Constant  Value=0.0  OutDataTypeStr=single
  Constan3 : Constant  Value=40  OutDataTypeStr=single
  Constan4 : Constant  Value=0.0000024166  OutDataTypeStr=single
  Constan5 : Constant  Value=60  OutDataTypeStr=single
  Constan6 : Constant  Value=30000  OutDataTypeStr=single
  Constan7 : Constant  Value=3  OutDataTypeStr=single
  Constan8 : Constant  Value=3  OutDataTypeStr=single
  Constan9 : Constant  Value=60  OutDataTypeStr=single
  Constant2 : Constant  Value=Fmc_tiTFuelMassCorr
  Constant4 : Constant  Value=Fmc_facKFuelMassCorr
  Constant6 : Constant  Value=Fmc_flgFuelMassOverride
  Constant7 : Constant  Value=Fmc_flgFuelMassCorrEnable
  Constant8 : Constant  Value=Fmc_mFuelMan
  DT1 : Subsystem
      mask Description: DT1
      mask Display: image(imread('DT1.jpg'))
  DT1_Fcn : Subsystem
      mask Description: DT1_Fcn
      mask Display: image(imread('DT1.jpg'))
  Divide{,1..3} (4 alike) : Product  Inputs=*/  OutDataTypeStr=Inherit: Same as first input
  Fmc_mFuelKgPerHour : Terminator
  Fmc_specific_fuel_consumption : Terminator
  Manual Switch : simulink/Signal Routing/Manual Switch  sw=1  action=0  varsize=off
  MinMax : MinMax  Function=max  Inputs=2
  Product1 : Product  OutDataTypeStr=Inherit: Same as first input
  Product2 : Product  OutDataTypeStr=Inherit: Same as first input
  Product3 : Product  Inputs=4  OutDataTypeStr=Inherit: Same as first input
  Product4 : Product  Inputs=4  OutDataTypeStr=Inherit: Same as first input
  Product5 : Product  Inputs=3  OutDataTypeStr=Inherit: Same as first input
  Subtract : Sum  OutDataTypeStr=Inherit: Same as first input
  Subtract1 : Sum  OutDataTypeStr=Inherit: Same as first input
  Switch2 : Switch  Threshold=1
  Fmc_mFuel : Outport
  wires:
  Constant6/1 -> Switch2/2
  DT1/1(Out) -> Manual Switch/1  "Fmc_mFuelCorr"
  Constant2/1 -> DT1/1(T)
  Constant4/1 -> DT1/2(K)
  Constant7/1 -> DT1/6(Enable), DT1_Fcn/3(Enable)
  Constan3/1 -> Divide/1
  Divide/1 -> DT1/3(Ta)  "Fmc_tiTaFuelMassCorr"
  Constan2/1 -> DT1/5(initValue), DT1_Fcn/2(initValue)
  MinMax/1 -> Divide/2
  Epm_rpmEngSpd/1 -> MinMax/1, Product4/2
  Constan1/1 -> MinMax/2
  Amf_mAirPerStr/1 -> Divide1/1
  Afr_facRatio/1 -> Divide1/2
  Divide1/1 -> Subtract/2, DT1/4(in), DT1_Fcn/1(In)  "Fmc_mFuelBase"
  Constant8/1 -> Switch2/1
  Manual Switch/1 -> Subtract/1
  Subtract/1 -> Product1/1
  Lcc_facLambdaCorr/1 -> Product1/2
  Itc_tiInjOffset/1 -> Product2/1
  Product2/1 -> Subtract1/2
  Product1/1 -> Switch2/3  "Fmc_mFuelCalc"
  Switch2/1 -> Fmc_mFuel/1, Subtract1/1  "Fmc_mFuel"
  Constan4/1 -> Product2/2
  Subtract1/1 -> Product3/1, Product4/1
  Constan5/1 -> Product3/2
  Constan6/1 -> Product3/3
  Constan7/1 -> Product3/4
  Constan8/1 -> Product4/3
  Constan9/1 -> Product4/4
  Product4/1 -> Divide2/1
  Constan10/1 -> Divide2/2
  Constan12/1 -> Product5/1
  Tqs_tqReq/1 -> Product5/2
  Constan11/1 -> Product5/3
  Product3/1 -> Divide3/1
  Product5/1 -> Divide3/2
  Divide3/1 -> Fmc_specific_fuel_consumption/1  "Fmc_specific_fuel_consumption"
  Divide2/1 -> Fmc_mFuelKgPerHour/1  "Fmc_mFuelKgPerHour"
  DT1_Fcn/1(Out) -> Manual Switch/2  "Fmc_mFuelCorr_Fcn"

== system M160_lib/Functions/ICC_1 ==
  Mpc_pManiFilt : Inport
  function : TriggerPort  TriggerType=function-call
  Constant1 : Constant  Value=ICC_atManiOff
  Constant3 : Constant  Value=ICC_atManiOn
  RSFlipFlop : Subsystem
      mask Description: RSFlipFlop
      mask Display: image(imread('RSFlipFlop.jpg'))
  Relational Operator1 : RelationalOperator  Operator=<=  OutDataTypeStr=boolean
  Relational Operator2 : RelationalOperator  OutDataTypeStr=boolean
  Terminator : Terminator
  ICC_flgInterCooler : Outport
  wires:
  Mpc_pManiFilt/1 -> Relational Operator2/1, Relational Operator1/1
  Constant3/1 -> Relational Operator2/2
  Constant1/1 -> Relational Operator1/2
  RSFlipFlop/1(q) -> ICC_flgInterCooler/1  "ICC_flgInterCooler"
  RSFlipFlop/2(nq) -> Terminator/1
  Relational Operator2/1 -> RSFlipFlop/1(s)
  Relational Operator1/1 -> RSFlipFlop/2(r)

== system M160_lib/Functions/Iac ==
  note: Zündwinkelanpassung im Leerlauf:
      | Ist der Leerlaufregler aktiv wird aus dem schnellen Saugrohrdruckanteil und dem Ist-Saugrohrdruck
      | der Quotient gebildet. Aus diesem und mit Hilfe des Zündwinkelwirkungsgradkennfeldes wird ein
      | Delta-Zündwinkel ermittelt der auf den optimalen Zündwinkel addiert wird.
  Epm_rpmEngSpd : Inport
  Amf_facRelAir : Inport  Port=2
  Mpc_pManiFilt : Inport  Port=3
  Isc_flgIdleSpdCtrlActive : Inport  Port=4
  T2t_pManiReqFast : Inport  Port=5
  Stc_flgCatalyserHeating : Inport  Port=6
  function : TriggerPort  TriggerType=function-call
  Constan1 : Constant  Value=0.7  OutDataTypeStr=single
  Constan11 : Constant  Value=0.2  OutDataTypeStr=single
  Constan2 : Constant  Value=1.0  OutDataTypeStr=single
  Constan3 : Constant  Value=0.0  OutDataTypeStr=single
  Constant1 : Constant  Value=Iac_degIgnOptOffset
  Constant2 : Constant  Value=Iac_pManiReqMin
  Constant8 : Constant  Value=Iac_flgIgnCutoffReq
  Divide1 : Product  Inputs=*/  OutDataTypeStr=Inherit: Same as first input
  Iac_deltaDegIgn : Lookup_n-D  NumberOfTableDimensions=1  BreakpointsForDimension1=Iac_deltaDegIgn_x  Table=Iac_deltaDegIgn_y  ExtrapMethod=Clip  InputSameDT=on
  Iac_rpmEngSpdfacRelAir2degBase_MAP : Lookup_n-D  BreakpointsForDimension1=Iac_rpmEngSpdfacRelAir2degBase_MAP_x  BreakpointsForDimension2=Iac_rpmEngSpdfacRelAir2degBase_MAP_y  Table=Iac_rpmEngSpdfacRelAir2degBase_MAP_z  ExtrapMethod=Clip  InputSameDT=on
  Iac_rpmEngSpdfacRelAir2degMinAdvBestTq_MAP : Lookup_n-D  BreakpointsForDimension1=Iac_rpmEngSpdfacRelAir2degMinAdvBestTq_MAP_x  BreakpointsForDimension2=Iac_rpmEngSpdfacRelAir2degMinAdvBestTq_MAP_y  Table=Iac_rpmEngSpdfacRelAir2degMinAdvBestTq_MAP_z  ExtrapMethod=Clip  InputSameDT=on
  Logical Operator3 : Logic  Operator=OR  AllPortsSameDT=off  OutDataTypeStr=boolean
  MinMax : MinMax  Function=max  Inputs=2
  MinMax1 : MinMax  Inputs=2
  Subtract1 : Sum  Inputs=+-  OutDataTypeStr=Inherit: Same as first input
  Subtract2 : Sum  Inputs=+-  OutDataTypeStr=Inherit: Same as first input
  Subtract3 : Sum  OutDataTypeStr=Inherit: Same as first input
  Subtract4 : Sum  Inputs=+-  OutDataTypeStr=Inherit: Same as first input
  Switch1 : Switch  Threshold=1
  Switch2 : Switch  Threshold=1
  Iac_flgIgnCutoff : Outport
  Iac_degIgnIdleSpeed : Outport  Port=2
  Iac_degIgn : Outport  Port=3
  Iac_degMinAdvBestTq : Outport  Port=4
  wires:
  Constant8/1 -> Iac_flgIgnCutoff/1  "Iac_flgIgnCutoff"
  Constant1/1 -> Subtract3/1
  Iac_rpmEngSpdfacRelAir2degBase_MAP/1 -> Subtract3/2  "Iac_degIgnBase"
  Epm_rpmEngSpd/1 -> Iac_rpmEngSpdfacRelAir2degBase_MAP/1, Iac_rpmEngSpdfacRelAir2degMinAdvBestTq_MAP/1
  Amf_facRelAir/1 -> Iac_rpmEngSpdfacRelAir2degBase_MAP/2, Iac_rpmEngSpdfacRelAir2degMinAdvBestTq_MAP/2
  Constan1/1 -> Switch1/3
  Stc_flgCatalyserHeating/1 -> Switch1/2, Logical Operator3/2
  Constan11/1 -> Switch1/1
  Switch1/1 -> MinMax/1
  T2t_pManiReqFast/1 -> Subtract1/1
  Subtract1/1 -> Divide1/1
  Constant2/1 -> Subtract1/2, Subtract2/2
  Mpc_pManiFilt/1 -> Subtract2/1
  Subtract2/1 -> Divide1/2
  MinMax1/1 -> MinMax/2
  Divide1/1 -> MinMax1/1
  Constan2/1 -> MinMax1/2
  Iac_rpmEngSpdfacRelAir2degMinAdvBestTq_MAP/1 -> Iac_degMinAdvBestTq/1  "Iac_degMinAdvBestTq"
  Subtract3/1 -> Iac_degIgn/1, Subtract4/1  "Iac_degIgn"
  Subtract4/1 -> Iac_degIgnIdleSpeed/1  "Iac_degIgnIdleSpeed"
  Isc_flgIdleSpdCtrlActive/1 -> Logical Operator3/1
  Logical Operator3/1 -> Switch2/2
  Switch2/1 -> Subtract4/2
  Iac_deltaDegIgn/1 -> Switch2/1
  Constan3/1 -> Switch2/3
  MinMax/1 -> Iac_deltaDegIgn/1
